simulink model "DigitalShadow"  (R2022a)
settings: Solver=FixedStepDiscrete  StartTime=0.0  StopTime=4  FixedStep=ControlPeriod/10  MaxStep=ControlPeriod/10  RelTol=1e-3
InitFcn:
  | Emrax_params;
model workspace (MAT data in the model file):
  CTRLPERIOD = 5e-05
  TSAMPLE = 2e-06
  global_CLK_number = 0
  global_INT_number = 1
  global_SVM_instance_id = 0
  global_can_baud_rate = '1000000'
  global_comp_time = 0.2
  global_cycle_delay = 0
  global_ip_addresses = {'10.10.10.110', '10.10.10.111', '10.10.10.112', '10.10.10.113'}
values from neighbouring files (symbols this model uses):
  ControlPeriod = 1/ControlFreq    (= 5e-05)    [Emrax_params.m]
  fc_s = 5    [Emrax_params.m]
  PI_d = pidtune(Hd,'PI',2*pi*f_i,opts)    [Emrax_params.m]
  PI_q = pidtune(Hq,'PI',2*pi*f_i,opts)    [Emrax_params.m]
  PI_s = pidtune(Hs,'PI',2*pi*fc_s,opts)    [Emrax_params.m]
  Vdc0 = 400    [Emrax_params.m]
undefined symbols (not defined in the file or in its folder): DiscIntNeverNeededParam, Pmsm
libraries: spsPWMGenerator2LevelLib x3, simulink x2, BoomBox x1, spsabctodq0Lib x1, spsdq0toabcLib x1, spsCurrentMeasurementLib x1, spsDCVoltageSourceLib x1, spsPermanentMagnetSynchronousMachineLib x1, spsThreePhaseSeriesRLCBranchLib x1, spsThreePhaseVIMeasurementLib x1, spsUniversalBridgeLib x1, spsVoltageMeasurementLib x1
settings Model: TunableVars=MODE  TunableVarsStorageClass=ImportedExtern  Creator=imperix  LastModifiedBy=JHANNUM
settings SolverCC: AlgebraicLoopSolver=TrustRegion
settings DataIOCC: LimitDataPoints=on  SaveFormat=Array  SaveOutput=off  SaveTime=off  ReturnWorkspaceOutputs=off
settings OptimizationCC: DefaultUnderspecifiedDataType=single  EnhancedBackFolding=on  PassReuseOutputArgsAs=Individual arguments  ZeroExternalMemoryAtStartup=off  ZeroInternalMemoryAtStartup=off  LifeSpan=inf  SimCompilerOptimization=on  EfficientTunableParamExpr=on
settings DebuggingCC: UnderspecifiedInitializationDetection=Classic  InheritedTsInSrcMsg=none  ParameterPrecisionLossMsg=none  ParameterTunabilityLossMsg=error  UnconnectedInputMsg=warning  UnconnectedOutputMsg=warning  UnconnectedLineMsg=warning  SFUnexpectedBacktrackingDiag=warning  SFNoUnconditionalDefaultTransitionDiag=warning  SFMachineParentedDataDiag=warning  ArithmeticOperatorsInVariantConditions=warning
settings HardwareCC: ProdBitPerPointer=32  ProdBitPerSizeT=32  ProdBitPerPtrDiffT=32  ProdLargestAtomicInteger=Long  ProdLargestAtomicFloat=Double  ProdWordSize=32  ProdHWDeviceType=ARM Compatible->ARM Cortex
settings ModelReferenceCC: UpdateModelReferenceTargets=IfOutOfDate  PropagateSignalLabelsOutOfModel=off
settings SFSimCC: SFSimEcho=off  SimUseLocalCustomCode=off  MATLABDynamicMemAlloc=off  CustomCodeUndefinedFunction=UseInterfaceOnly  SimTargetLang=C++
settings RTWCC: Description=Embedded Coder for imperix products  SystemTargetFile=imperix_ACG_SDK.tlc  TemplateMakefile=imperix_ACG_SDK.tmf  RTWUseLocalCustomCode=off  RTWUseSimCustomCode=on  TargetLang=C++  RTWCustomCompilerOptimizations=-a  DLArmComputeVersion=19.05
settings CodeAppCC: ForceParamTrailComments=on  IgnoreCustomStorageClasses=off  OperatorAnnotations=on  SimulinkDataObjDesc=on  SFDataObjDesc=on  InsertBlockDesc=on  StateflowObjectComments=on
settings STFCustomTargetCC: MultiwordLength=256  ModelReferenceCompliant=off  CombineOutputUpdateFcns=on  ERTCustomFileBanners=on  SupportContinuousTime=off  SupportNonInlinedSFcns=off  RemoveResetFunc=on  MATLABClassNameForMDSCustomization=Simulink.SoftwareTarget.ERTCustomization  GRTInterface=off  SystemTargetFile=imperix_ACG_SDK.tlc
settings ERTTargetCC: ModelReferenceCompliant=off  ParMdlRefBuildCompliant=off  CompOptLevelCompliant=off  ConcurrentExecutionCompliant=off  ModelStepFunctionPrototypeControlCompliant=off  CPPClassGenCompliant=off  UseToolchainInfoCompliant=off  ExtModeStaticAlloc=on  ExtModeStaticAllocSize=100000  ERTSrcFileBannerTemplate=imperix_ACG_SDK_code_template.cgt  ERTHdrFileBannerTemplate=imperix_ACG_SDK_code_template.cgt  ERTDataSrcFileTemplate=imperix_ACG_SDK_code_template.cgt  ERTDataHdrFileTemplate=imperix_ACG_SDK_code_template.cgt  ERTCustomFileTemplate=imperix_ACG_SDK_file_process.tlc  MemSecPackage=Simulink
settings ConfigComp: CovMetricSettings=dw  CovSaveCumulativeToWorkspaceVar=on  CovSaveSingleToWorkspaceVar=on  CovExternalEMLEnable=off
settings SimscapeCC: SimscapeNormalizeSystem=off

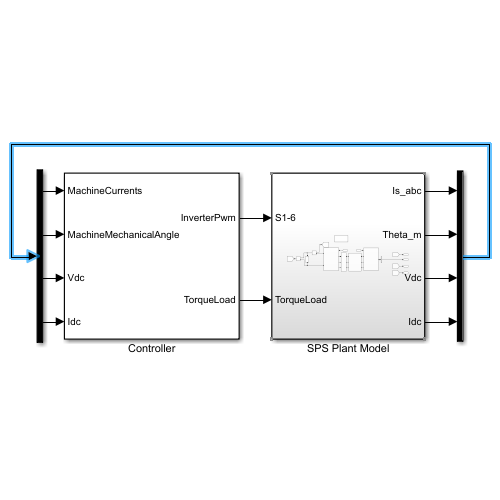
[thumbnail: Simulink's stored preview of the top-level diagram]
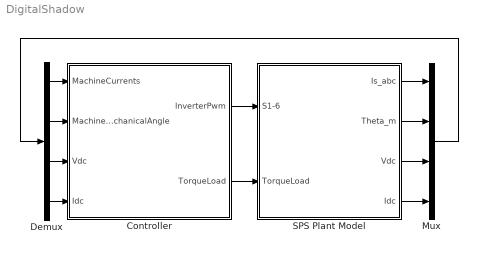
== system DigitalShadow ==
  Controller : Subsystem
  Demux : Demux  Outputs=[3 1 1 1]
  Mux : Mux  Inputs=[3 1 1 1]
  SPS Plant Model : Subsystem
  wires:
  Controller/1(InverterPwm) -> SPS Plant Model/1(S1-6)
  Demux/2 -> Controller/2(MachineMechanicalAngle)
  SPS Plant Model/2(Theta_m) -> Mux/2
  Demux/1 -> Controller/1(MachineCurrents)
  SPS Plant Model/1(Is_abc) -> Mux/1
  SPS Plant Model/3(Vdc) -> Mux/3
  SPS Plant Model/4(Idc) -> Mux/4
  Demux/3 -> Controller/3(Vdc)
  Demux/4 -> Controller/4(Idc)
  Mux/1 -> Demux/1
  Controller/2(TorqueLoad) -> SPS Plant Model/2(TorqueLoad)

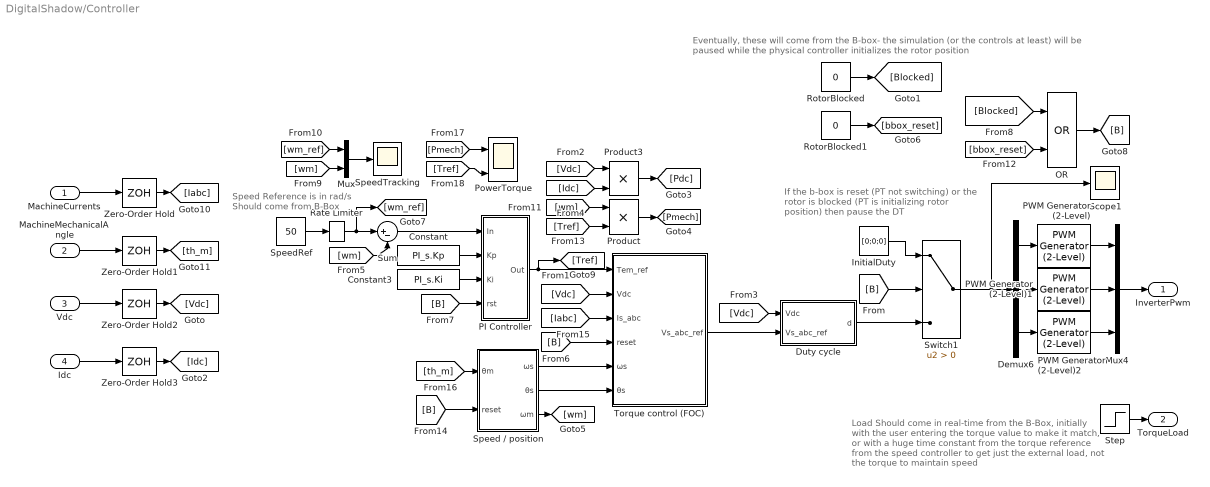
== system DigitalShadow/Controller ==
  note: Speed Reference is in rad/s
      | Should come from B-Box
  note: If the b-box is reset (PT not switching) or the rotor is blocked (PT is initializing rotor position) then pause the DT
  note: Eventually, these will come from the B-box- the simulation (or the controls at least) will be paused while the physical controller initializes the rotor position
  note: Load Should come in real-time from the B-Box, initially with the user entering the torque value to make it match, or with a huge time constant from the torque reference from the speed controller to get just the external load, not the torque to maintain speed
  MachineCurrents : Inport
  MachineMechanicalAngle : Inport  Port=2
  Vdc : Inport  Port=3
  Idc : Inport  Port=4
  Constant : Constant  Value=PI_s.Kp  SampleTime=ControlPeriod
  Constant3 : Constant  Value=PI_s.Ki  SampleTime=ControlPeriod
  Demux6 : Demux  Outputs=3
  Duty cycle : Subsystem
  InitialDuty : Constant  Value=[0;0;0]  SampleTime=ControlPeriod
  Mux : Mux  Inputs=2
  Mux4 : Mux  Inputs=3
  OR : Logic  Operator=OR  IconShape=distinctive  AllPortsSameDT=off  OutDataTypeStr=boolean
  PI Controller : Subsystem  mask(PI controller){I_MODE=Trapezoidal, SamplingTime=ControlPeriod, S_MODE=on, SaturationUpperLimit=100, SaturationLowerLimit=-100, LinearizeAsGain=off, ANTI_WINDUP=back-calculation, K_B=0.1*sqrt(PI_s.Kp*PI_s.Ki)}
      mask prompts: S_MODE "Limit output"; LinearizeAsGain "Ignore saturation when linearizing"
      mask help: This subsystem implements a Proportional Integral (PI) controller, as described in the Technical Note T105.
      mask init:
      | thisBlock = gcb;
      | 
      | 
      | 
      | % change the integrator mode depending on the radio button
      | tempBlock = [gcb '/Integrator'];
      | int_mode = get_param(thisBlock, 'I_MODE')
      | if strcmp('Forward Euler', int_mode)
      |     set_param(tempBlock,'IntegratorMethod','Integration: Forward Euler' )  
      | elseif strcmp('Backward Euler', int_mode)
      |     set_param(tempBlock,'IntegratorMethod','Integration: Backward Euler')  
      | else
      |     set_param(tempBlock,'IntegratorMethod','Integration: Trapezoidal' )  
      | end
      | 
      | 
      | % change the parameters in the saturation block
      | tempBlock = [gcb '/Saturation'];
      | if strcmp('on', get_param(gcb, 'S_MODE'))
      |     set_param(tempBlock, 'OverrideUsingVariant', 'WITH_SATURATION'); 
      | else
      |     set_param(tempBlock, 'OverrideUsingVariant', 'WITHOUT_SATURATION'); 
      | end
      | tempBlock = [gcb '/Saturation/With saturation/Saturation'];
      | set_param(tempBlock, 'UpperLimit', get_param(thisBlock, 'SaturationUpperLimit')); 
      | set_param(tempBlock, 'LowerLimit', get_param(thisBlock, 'SaturationLowerLimit')); 
      | set_param(tempBlock, 'LinearizeAsGain', get_param(thisBlock, 'LinearizeAsGain')); 
      | 
      | 
      | 
      | % change the anti-windup
      | tempBlock = [gcb '/Anti-windup'];
      | if strcmp('none', get_param(thisBlock, 'ANTI_WINDUP'))
      |     set_param(tempBlock, 'OverrideUsingVariant', 'WITHOUT_ANTI_WINDUP'); 
      | else
      |     set_param(tempBlock, 'OverrideUsingVariant', 'WITH_ANTI_WINDUP'); 
      | end
      | tempBlock = [gcb '/Anti-windup/With anti-windup/Kb'];
      | set_param(tempBlock, 'Gain', get_param(thisBlock, 'K_B')); 
      | 
      | clear thisBlock tempBlock
      mask TypeOptions I_MODE: Forward Euler | Backward Euler | Trapezoidal
      mask Callback I_MODE:
      | thisBlock = gcb;
      | tempBlock = [gcb '/Integrator'];
      | 
      | % change the integrator mode depending on the radio button:
      | int_mode = get_param(thisBlock, 'I_MODE')
      | if strcmp('Forward Euler', int_mode)
      |     set_param(tempBlock,'IntegratorMethod','Integration: Forward Euler' )
      | elseif strcmp('Backward Euler', int_mode)
      |     set_param(tempBlock,'IntegratorMethod','Integration: Backward Euler')
      | else
      |     set_param(tempBlock,'IntegratorMethod','Integration: Trapezoidal' )
      | end
      | 
      | clear thisBlock tempBlock;
      mask Callback S_MODE:
      | thisBlock = gcb;
      | tempBlock = [gcb '/Saturation'];
      | 
      | % change the saturation mode depending on the radio button:
      | if strcmp('on', get_param(gcb, 'S_MODE'))
      |     set_param(tempBlock, 'OverrideUsingVariant', 'WITH_SATURATION');
      | else
      |     set_param(tempBlock, 'OverrideUsingVariant', 'WITHOUT_SATURATION');
      | end
      | 
      | % Hide or show parameters
      | maskNames = get_param(thisBlock, 'MaskNames');
      | maskEnable = get_param(thisBlock, 'MaskEnables');
      | 
      | if strcmp(get_param(thisBlock, 'S_MODE'),'on')
      |     %show parameters
      |     maskEnable{strmatch('SaturationUpperLimit',  maskNames, 'exact')} = 'on';
      |     maskEnable{strmatch('SaturationLowerLimit',   maskNames, 'exact')} = 'on';
      |     maskEnable{strmatch('LinearizeAsGain',   maskNames, 'exact')} = 'on';
      |     maskEnable{strmatch('ANTI_WINDUP',   maskNames, 'exact')} = 'on';
      |     maskEnable{strmatch('K_B',   maskNames, 'exact')} = 'on';
      | else
      |     %hide parameters
      |     maskEnable{strmatch('SaturationUpperLimit',  maskNames, 'exact')} = 'off';
      |     maskEnable{strmatch('SaturationLowerLimit',   maskNames, 'exact')} = 'off';
      |     maskEnable{strmatch('LinearizeAsGain',   maskNames, 'exact')} = 'off';
      |     maskEnable{strmatch('ANTI_WINDUP',   maskNames, 'exact')} = 'off';
      |     maskEnable{strmatch('K_B',   maskNames, 'exact')} = 'off';
      | end
      | 
      | set_param(thisBlock, 'MaskEnables', maskEnable);
      | 
      | clear thisBlock tempBlock maskNames maskEnable;
      mask Callback SaturationUpperLimit:
      | thisBlock = gcb;
      | tempBlock = [gcb '/Saturation/With saturation/Saturation'];
      | 
      | % change the parameter in the subblock
      | set_param(tempBlock, 'UpperLimit', get_param(thisBlock, 'SaturationUpperLimit'));
      | 
      | clear thisBlock tempBlock
      mask Callback SaturationLowerLimit:
      | thisBlock = gcb;
      | tempBlock = [gcb '/Saturation/With saturation/Saturation'];
      | 
      | % change the parameter in the subblock
      | set_param(tempBlock, 'LowerLimit', get_param(thisBlock, 'SaturationLowerLimit'));
      | 
      | clear thisBlock tempBlock
      mask Callback LinearizeAsGain:
      | thisBlock = gcb;
      | tempBlock = [gcb '/Saturation/With saturation/Saturation'];
      | 
      | % change the parameter in the subblock
      | set_param(tempBlock, 'LinearizeAsGain', get_param(thisBlock, 'LinearizeAsGain'));
      | 
      | clear thisBlock tempBlock
      mask TypeOptions ANTI_WINDUP: none | back-calculation
      mask Callback ANTI_WINDUP:
      | thisBlock = gcb;
      | tempBlock = [gcb '/Anti-windup'];
      | 
      | % change the saturation mode depending on the radio button:
      | if strcmp('none', get_param(thisBlock, 'ANTI_WINDUP'))
      |     set_param(tempBlock, 'OverrideUsingVariant', 'WITHOUT_ANTI_WINDUP');
      | else
      |     set_param(tempBlock, 'OverrideUsingVariant', 'WITH_ANTI_WINDUP');
      | end
      | 
      | % Hide or show parameters
      | maskNames = get_param(thisBlock, 'MaskNames');
      | MaskVisibility = get_param(thisBlock, 'MaskVisibilities');
      | 
      | if strcmp(get_param(thisBlock, 'ANTI_WINDUP'),'none')
      |     %hide parameters
      |     MaskVisibility{strmatch('K_B',  maskNames, 'exact')} = 'off';
      |     %thisBlock.getDialogControl('KBtext').Visible='off';
      | else
      |     %show parameters
      |     MaskVisibility{strmatch('K_B',  maskNames, 'exact')} = 'on';
      |     %thisBlock.getDialogControl('KBtext').Visible='on';
      | end
      | 
      | set_param(thisBlock, 'MaskVisibilities', MaskVisibility);
      | 
      | clear thisBlock tempBlock maskNames MaskVisibility;
      mask Callback K_B:
      | thisBlock = gcb;
      | tempBlock = [gcb '/Anti-windup/With anti-windup/Kb'];
      | 
      | % change the parameter in the subblock
      | set_param(tempBlock, 'Gain', get_param(thisBlock, 'K_B'));
      | 
      | clear thisBlock tempBlock
      mask DialogControl DiscreteText Prompt: Discrete-time settings
      mask DialogControl I_MODEText Prompt: Integrator method:
      mask DialogControl SamplingTimeText Prompt: Sample time (-1 for inherited)
      mask DialogControl SaturationText Prompt: Output saturation
      mask DialogControl Control4 Prompt: Upper saturation limit:
      mask DialogControl Control5 Prompt: Lower saturation limit:
      mask DialogControl Control6 Prompt: Anti-windup method:
      mask DialogControl KBtext Prompt: Back-calculation coefficient (Kb):
  PWM Generator (2-Level) : spsPWMGenerator2LevelLib/PWM Generator (2-Level)  ModulatorType=Single-phase half-bridge (2 pulses)  ModulatorMode=Unsynchronized  Fc=ControlFreq  Pc=0  nF=1  MinMax=[0 1]  SamplingTechnique=Symmetrical regular (single edge)  ModulatingSignals=off  m=0.8  Freq=60  Phase=0  Ts=ControlPeriod/10  ShowCarrierOutport=off
  PWM Generator (2-Level)1 : spsPWMGenerator2LevelLib/PWM Generator (2-Level)  ModulatorType=Single-phase half-bridge (2 pulses)  ModulatorMode=Unsynchronized  Fc=ControlFreq  Pc=0  nF=1  MinMax=[0 1]  SamplingTechnique=Symmetrical regular (single edge)  ModulatingSignals=off  m=0.8  Freq=60  Phase=0  Ts=ControlPeriod/10  ShowCarrierOutport=off
  PWM Generator (2-Level)2 : spsPWMGenerator2LevelLib/PWM Generator (2-Level)  ModulatorType=Single-phase half-bridge (2 pulses)  ModulatorMode=Unsynchronized  Fc=ControlFreq  Pc=0  nF=1  MinMax=[0 1]  SamplingTechnique=Symmetrical regular (single edge)  ModulatingSignals=off  m=0.8  Freq=60  Phase=0  Ts=ControlPeriod/10  ShowCarrierOutport=off
  PowerTorque : Scope  NumInputPorts=2
  Product : Product
  Product3 : Product
  Rate Limiter : RateLimiter  RisingSlewLimit=100  FallingSlewLimit=-25  SampleTimeMode=inherited  LinearizeAsGain=off
  RotorBlocked : Constant  Value=0  SampleTime=ControlPeriod
  RotorBlocked1 : Constant  Value=0  SampleTime=ControlPeriod
  Scope1 : Scope
  Speed / position : Subsystem
  SpeedRef : Constant  Value=50  SampleTime=ControlPeriod
  SpeedTracking : Scope
  Step : Step  After=10  SampleTime=ControlPeriod
  Sum : Sum  Inputs=|+-
  Switch1 : Switch  Criteria=u2 > Threshold  SaturateOnIntegerOverflow=off  InputSameDT=off
  Torque control (FOC) : Subsystem
  Zero-Order Hold{,1..3} (4 alike) : ZeroOrderHold  SampleTime=ControlPeriod
  InverterPwm : Outport
  TorqueLoad : Outport  Port=2
  wires:
  PWM Generator (2-Level)1/1 -> Mux4/2
  PWM Generator (2-Level)/1 -> Mux4/1
  PWM Generator (2-Level)2/1 -> Mux4/3
  [Vdc] -> Torque control (FOC)/2(Vdc)
  Speed / position/2(θs) -> Torque control (FOC)/6(θs)
  Torque control (FOC)/1(Vs_abc_ref) -> Duty cycle/2(Vs_abc_ref)
  [Vdc] -> Duty cycle/1(Vdc)
  Sum/1 -> PI Controller/1(In)
  Speed / position/3(" ωm") -> [wm]
  Mux4/1 -> InverterPwm/1
  Duty cycle/1(d) -> Switch1/3
  Switch1/1 -> Scope1/1, Demux6/1
  [B] -> Switch1/2
  PI Controller/1(Out) -> Torque control (FOC)/1(Tem_ref), [Tref]
  [B] -> Torque control (FOC)/4(reset)
  [B] -> PI Controller/4(rst)
  Rate Limiter/1 -> [wm_ref], Sum/1
  [B] -> Speed / position/2(reset)
  Speed / position/1(" ωs") -> Torque control (FOC)/5(ωs)
  Product/1 -> [Pmech]
  [Vdc] -> Product3/1
  [Idc] -> Product3/2
  Product3/1 -> [Pdc]
  SpeedRef/1 -> Rate Limiter/1
  Demux6/3 -> PWM Generator (2-Level)2/1
  Demux6/1 -> PWM Generator (2-Level)/1
  Demux6/2 -> PWM Generator (2-Level)1/1
  [wm] -> Sum/2
  Constant3/1 -> PI Controller/3(Ki)
  Constant/1 -> PI Controller/2(Kp)
  [wm] -> Mux/2
  [wm_ref] -> Mux/1
  Mux/1 -> SpeedTracking/1
  [wm] -> Product/1
  InitialDuty/1 -> Switch1/1
  RotorBlocked1/1 -> [bbox_reset]
  [Blocked] -> OR/1
  [bbox_reset] -> OR/2
  OR/1 -> [B]
  [Tref] -> Product/2
  [Iabc] -> Torque control (FOC)/3(Is_abc)
  [th_m] -> Speed / position/1(θm)
  Zero-Order Hold/1 -> [Iabc]
  Zero-Order Hold1/1 -> [th_m]
  Zero-Order Hold2/1 -> [Vdc]
  Zero-Order Hold3/1 -> [Idc]
  RotorBlocked/1 -> [Blocked]
  [Pmech] -> PowerTorque/1
  [Tref] -> PowerTorque/2
  MachineCurrents/1 -> Zero-Order Hold/1
  MachineMechanicalAngle/1 -> Zero-Order Hold1/1
  Vdc/1 -> Zero-Order Hold2/1
  Idc/1 -> Zero-Order Hold3/1
  Step/1 -> TorqueLoad/1

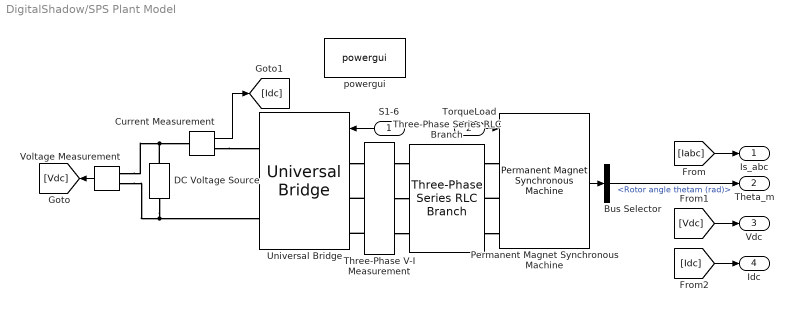
== system DigitalShadow/SPS Plant Model ==
  S1-6 : Inport
  TorqueLoad : Inport  Port=2
  Bus Selector : BusSelector  OutputSignals=Rotor angle thetam (rad)
  Current Measurement : spsCurrentMeasurementLib/Current Measurement  PhasorSimulation=off  OutputType=Complex  PSBequivalent=0
  DC Voltage Source : spsDCVoltageSourceLib/DC Voltage Source  Amplitude=Vdc0  Measurements=None
  Permanent Magnet Synchronous Machine : spsPermanentMagnetSynchronousMachineLib/Permanent Magnet Synchronous Machine  NbPhases=3  FluxDistribution=Sinusoidal  RotorType=Salient-pole  MechanicalLoad=Torque Tm  PresetModel=No  ShowDetailedParameters=on  MeasurementBus=off  Resistance=Pmsm.Rs  Inductance=8.5e-3  dqInductances=[76e-6,79e-6]  La=0.000395  MachineConstant=Flux linkage established by magnets (V.s)  Flux=Pmsm.Phi_pm  VoltageCst=64.3899  TorqueCst=0.5325  Flat=120  Mechanical=[Pmsm.Jm 0 Pmsm.p 0]  PolePairs=4  InitialConditions=[0,0, 0,0]  InitialConditions5ph=[0 0 0 0 0 0]  RefAngle=Aligned with phase A axis (original Park)  IterativeDiscreteModel=Trapezoidal robust  TsBlock=ControlPeriod/100  TsPowergui=0
  Three-Phase Series RLC Branch : spsThreePhaseSeriesRLCBranchLib/Three-Phase Series RLC Branch  LConnTagsString=A|B|C  RConnTagsString=A|B|C  BranchType=L  Resistance=1  Inductance=Pmsm.Lext  Capacitance=1e-6  Measurements=None
  Three-Phase V-I Measurement : spsThreePhaseVIMeasurementLib/Three-Phase V-I Measurement  VoltageMeasurement=phase-to-phase  SetLabelV=on  LabelV=Vabc  Vpu=off  VpuLL=off  CurrentMeasurement=yes  SetLabelI=on  LabelI=Iabc  Ipu=off  Pbase=100e6  Vbase=500e3  OutputType=Complex  PhasorSimulation=off  PSBequivalent=0
  Universal Bridge : spsUniversalBridgeLib/Universal Bridge  Arms=3  SnubberResistance=1e5  SnubberCapacitance=inf  Device=MOSFET / Diodes  Ron=1e-3  Lon=0  ForwardVoltages="[  0  0  ]"  ForwardVoltage=0  GTOparameters=[ 10e-6 , 20e-6 ]  IGBTparameters=[ 1e-6 , 2e-6 ]  Measurements=None  Measurements_2=None  converterType=Rectifier
  Voltage Measurement : spsVoltageMeasurementLib/Voltage Measurement  PhasorSimulation=off  OutputType=Complex  PSBequivalent=0
  powergui : spspowerguiLib/powergui  Priority=1  SimulationMode=Discrete  SampleTime=ControlPeriod/10  frequency=60  Iterations=50  frequencyindice=0  Pbase=100e6  ErrMax=1e-4  UnitsV=kV  UnitsW=MW  buscounter=0  FunctionMessages=off  echomessages=off  EnableUseOfTLC=off  CurrentSourceSwitches=off  DisableSnubberDevices=off  DisableRonSwitches=off  DisableVfSwitches=off  DisplayEquations=off  AutomaticDiscreteSolvers=off  SolverType=Tustin/Backward Euler (TBE)  Interpol=off  ExternalGateDelay=off  methode=off  Ts=100  x0status=blocks  SPID=on  SwTol=0  HookPort=off  NonlinearTolerance=1e-4  nMaxIteration=100  ContinueOnMaxIteration=off  RestoreLinks=warning  ResistiveCurrentMeasurement=off  Frange=[0:2:500]  Ylog=off  Xlog=on  ShowGrid=off  save=off  variable=ZData  structure=0  ZoomFFT=off  StartTime=0.0  cycles=1  DisplayStyle=1  fundamental=60  FreqAxis=off  MaxFrequency=1000  frequencyindicesteady=1  RmsSteady=1  display=off
  Is_abc : Outport
  Theta_m : Outport  Port=2
  Vdc : Outport  Port=3
  Idc : Outport  Port=4
  wires:
  S1-6/1 -> Universal Bridge/1
  [Iabc] -> Is_abc/1
  Voltage Measurement/1 -> [Vdc]
  [Vdc] -> Vdc/1
  Current Measurement/1 -> [Idc]
  [Idc] -> Idc/1
  Permanent Magnet Synchronous Machine/1 -> Bus Selector/1
  Bus Selector/1 -> Theta_m/1  "<Rotor angle thetam (rad)>"
  TorqueLoad/1 -> Permanent Magnet Synchronous Machine/1
  connections:
  DC Voltage Source/LConn1 -- Voltage Measurement/LConn2 -- Universal Bridge/RConn2
  Three-Phase V-I Measurement/LConn3 -- Universal Bridge/LConn3
  Three-Phase V-I Measurement/LConn2 -- Universal Bridge/LConn2
  Universal Bridge/LConn1 -- Three-Phase V-I Measurement/LConn1
  Three-Phase V-I Measurement/RConn3 -- Three-Phase Series RLC Branch/LConn3
  Three-Phase V-I Measurement/RConn2 -- Three-Phase Series RLC Branch/LConn2
  Three-Phase V-I Measurement/RConn1 -- Three-Phase Series RLC Branch/LConn1
  Three-Phase Series RLC Branch/RConn1 -- Permanent Magnet Synchronous Machine/LConn1
  Permanent Magnet Synchronous Machine/LConn2 -- Three-Phase Series RLC Branch/RConn2
  Three-Phase Series RLC Branch/RConn3 -- Permanent Magnet Synchronous Machine/LConn3
  Voltage Measurement/LConn1 -- Current Measurement/LConn1 -- DC Voltage Source/RConn1
  Current Measurement/RConn1 -- Universal Bridge/RConn1

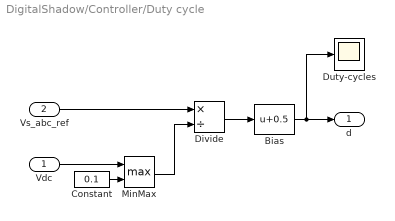
== system DigitalShadow/Controller/Duty cycle ==
  Vdc : Inport
  Vs_abc_ref : Inport  Port=2
  Bias : Bias  Bias=0.5  SaturateOnIntegerOverflow=off
  Constant : Constant  Value=0.1  OutDataTypeStr=single
  Divide : Product  Inputs=*/
  Duty-cycles : Scope
  MinMax : MinMax  Function=max  Inputs=2
  d : Outport
  wires:
  Vs_abc_ref/1 -> Divide/1
  Vdc/1 -> MinMax/1
  MinMax/1 -> Divide/2
  Constant/1 -> MinMax/2
  Divide/1 -> Bias/1
  Bias/1 -> Duty-cycles/1, d/1

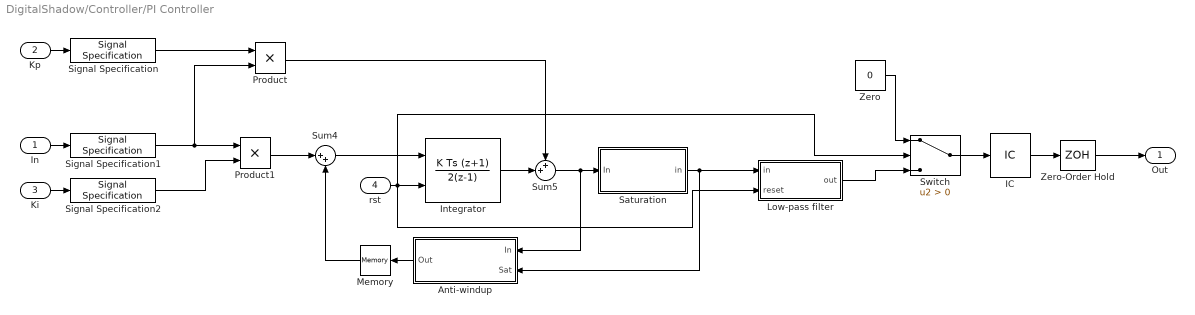
== system DigitalShadow/Controller/PI Controller ==
  In : Inport
  Kp : Inport  Port=2
  Ki : Inport  Port=3
  rst : Inport  Port=4
  Anti-windup : Subsystem  Variant=on  VariantControlMode=label  LabelModeActiveChoice=WITH_ANTI_WINDUP
  IC : InitialCondition  Value=0
  Integrator : DiscreteIntegrator  IntegratorMethod=Integration: Trapezoidal  ExternalReset=level  SampleTime=SamplingTime  ICPrevOutput=DiscIntNeverNeededParam  ICPrevScaledInput=DiscIntNeverNeededParam
  Low-pass filter : Subsystem
  Memory : Memory
  Product : Product
  Product1 : Product
  Saturation : Subsystem  Variant=on  VariantControlMode=label  LabelModeActiveChoice=WITH_SATURATION
  Signal Specification : SignalSpecification  SampleTime=SamplingTime
  Signal Specification1 : SignalSpecification  SampleTime=SamplingTime
  Signal Specification2 : SignalSpecification  SampleTime=SamplingTime
  Sum4 : Sum  Inputs=|++
  Sum5 : Sum  Inputs=++|
  Switch : Switch  Criteria=u2 > Threshold  SaturateOnIntegerOverflow=off  InputSameDT=off
  Zero : Constant  Value=0  OutDataTypeStr=Inherit: Inherit via back propagation
  Zero-Order Hold : ZeroOrderHold  SampleTime=CTRLPERIOD
  Out : Outport
  wires:
  Signal Specification2/1 -> Product1/2
  Signal Specification1/1 -> Product/2, Product1/1
  Signal Specification/1 -> Product/1
  Saturation/1(in) -> Low-pass filter/1(in), Anti-windup/2(Sat)
  Sum4/1 -> Integrator/1
  Kp/1 -> Signal Specification/1
  Product/1 -> Sum5/1
  Product1/1 -> Sum4/1
  Integrator/1 -> Sum5/2
  rst/1 -> Integrator/2, Low-pass filter/2(reset), Switch/2
  Sum5/1 -> Saturation/1(In), Anti-windup/1(In)
  In/1 -> Signal Specification1/1
  Ki/1 -> Signal Specification2/1
  Anti-windup/1(Out) -> Memory/1
  Memory/1 -> Sum4/2
  Switch/1 -> IC/1
  Zero/1 -> Switch/1
  IC/1 -> Zero-Order Hold/1
  Zero-Order Hold/1 -> Out/1
  Low-pass filter/1(out) -> Switch/3

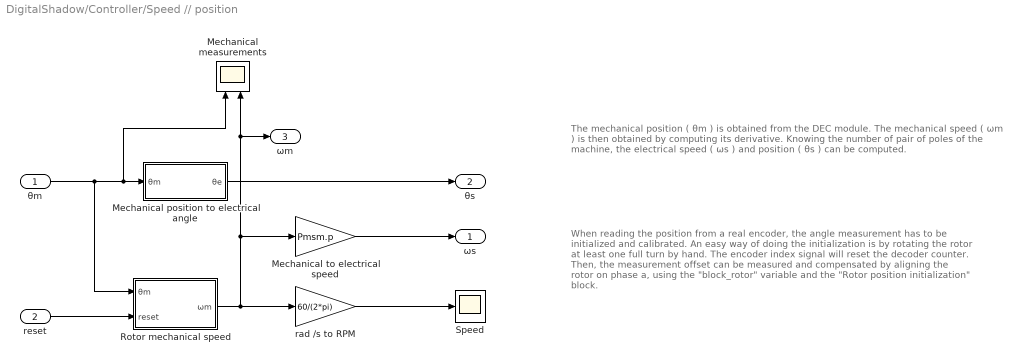
== system DigitalShadow/Controller/Speed // position ==
  note: The mechanical position ( θm ) is obtained from the DEC module.
      |
      | The mechanical speed ( ωm ) is then obtained by computing its derivative.
      |
      | Knowing the number of pair of poles of the machine, the electrical speed ( ωs ) and position ( θs ) can be computed.
  note: When reading the position from a real encoder, the angle measurement has to be initialized and calibrated.
      |
      | An easy way of doing the initialization is by rotating the rotor at least one full turn by hand. The encoder index signal will reset the decoder counter.
      |
      | Then, the measurement offset can be measured and compensated by aligning the rotor on phase a, using the "block_rotor" variable and the "Rotor position initialization" block.
  θm : Inport
  reset : Inport  Port=2
  Mechanical measurements : Scope  NumInputPorts=2
  Mechanical position to electrical angle : Subsystem  mask{p=Pmsm.p}
      mask prompts: p "Number of pole pairs"
  Mechanical to electrical speed : Gain  Gain=Pmsm.p
  Rotor mechanical speed : Subsystem  mask{fc=100}
      mask prompts: fc "Filter cutoff frequency [Hz]"
      mask help:
      | The rotor speed is obtained by differentiation of the measured angle. The "function block" removes angle discontinuities.
      |
      | The derivative is then filtered to reduce the noise introduced by the numerical differentiation.
      |
      | Additional details can be found in "PN104: Using the angle decoder modules" on the imperix knowledge base (kb.imperix.com).
  Speed : Scope
  rad /s to RPM : Gain  Gain=60/(2*pi)
  " ωs" : Outport
  θs : Outport  Port=2
  " ωm" : Outport  Port=3
  wires:
  reset/1 -> Rotor mechanical speed/2(reset)
  Mechanical position to electrical angle/1(θe) -> θs/1
  θm/1 -> Rotor mechanical speed/1(θm), Mechanical measurements/1, Mechanical position to electrical angle/1(θm)
  Rotor mechanical speed/1(ωm) -> rad /s to RPM/1, Mechanical to electrical speed/1, " ωm"/1, Mechanical measurements/2
  rad /s to RPM/1 -> Speed/1
  Mechanical to electrical speed/1 -> " ωs"/1

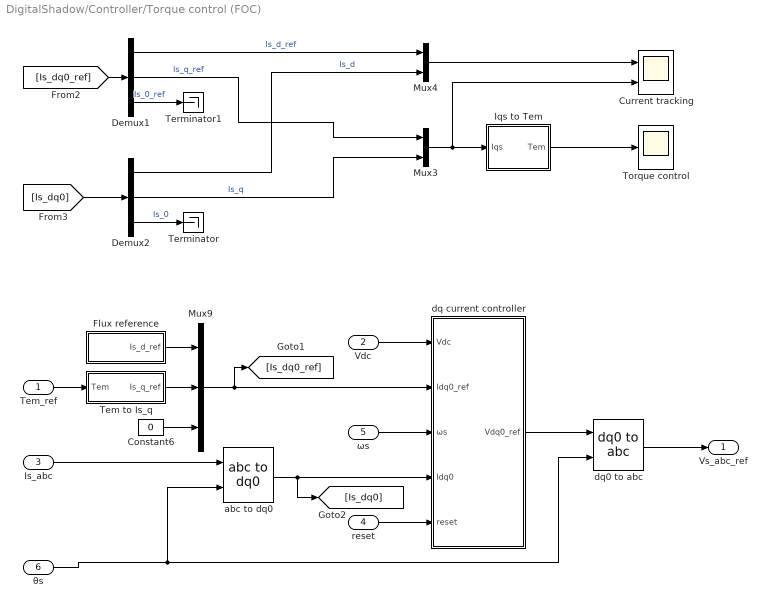
== system DigitalShadow/Controller/Torque control (FOC) ==
  Tem_ref : Inport
  Vdc : Inport  Port=2
  Is_abc : Inport  Port=3
  reset : Inport  Port=4
  ωs : Inport  Port=5
  θs : Inport  Port=6
  Constant6 : Constant  Value=0  OutDataTypeStr=Inherit: Inherit via back propagation
  Current tracking : Scope  NumInputPorts=2
  Demux1 : Demux  Outputs=3
  Demux2 : Demux  Outputs=3
  Flux reference : Subsystem
  Iqs to Tem : Subsystem  mask{p=Pmsm.p, Phi_pm=Pmsm.Phi_pm}
      mask prompts: p "Number of pole pairs"; Phi_pm "Magnets flux"
  Mux3 : Mux  Inputs=2
  Mux4 : Mux  Inputs=2
  Mux9 : Mux  Inputs=[1 1 1]
  Tem to Is_q : Subsystem  mask{p=Pmsm.p, Phi_pm=Pmsm.Phi_pm}
      mask prompts: p "Number of pole pairs"; Phi_pm "Permanent magnet flux [Wb]"
  Terminator : Terminator
  Terminator1 : Terminator
  Torque control : Scope
  abc to dq0 : spsabctodq0Lib/abc to dq0  Alignment=Aligned with phase A axis
  dq current controller : Subsystem  mask{Ld=Pmsm.Ld, Kpd=PI_d.Kp, Kid=PI_d.Ki, Lq=Pmsm.Lq, Kpq=PI_q.Kp, Kiq=PI_q.Ki}
      mask prompts: Ld "Inductance Ld"; Kpd "Proportional gain Kp"; Kid "Integral gain Ki"; Lq "Inductance Lq"; Kpq "Proportional gain Kp"; Kiq "Integral gain Ki"
      mask DialogControl ParameterGroupVar Prompt: Parameters: d-axis
      mask DialogControl Container3 Prompt: Parameters: q-axis
  dq0 to abc : spsdq0toabcLib/dq0 to abc  Alignment=Aligned with phase A axis
  Vs_abc_ref : Outport
  wires:
  Tem_ref/1 -> Tem to Is_q/1(Tem)
  Tem to Is_q/1(Is_q_ref) -> Mux9/2
  Flux reference/1(Is_d_ref) -> Mux9/1
  Constant6/1 -> Mux9/3
  dq0 to abc/1 -> Vs_abc_ref/1
  θs/1 -> dq0 to abc/2, abc to dq0/2
  abc to dq0/1 -> dq current controller/4(Idq0), [Is_dq0]
  reset/1 -> dq current controller/5(reset)
  Mux9/1 -> dq current controller/2(Idq0_ref), [Is_dq0_ref]
  dq current controller/1(Vdq0_ref) -> dq0 to abc/1
  Is_abc/1 -> abc to dq0/1
  Vdc/1 -> dq current controller/1(Vdc)
  Demux2/3 -> Terminator/1  "Is_0"
  Demux2/1 -> Mux4/2  "Is_d"
  Demux2/2 -> Mux3/2  "Is_q"
  Mux3/1 -> Current tracking/2, Iqs to Tem/1(Iqs)
  Mux4/1 -> Current tracking/1
  Iqs to Tem/1(Tem) -> Torque control/1
  Demux1/3 -> Terminator1/1  "Is_0_ref"
  Demux1/1 -> Mux4/1  "Is_d_ref"
  Demux1/2 -> Mux3/1  "Is_q_ref"
  [Is_dq0] -> Demux2/1
  [Is_dq0_ref] -> Demux1/1
  ωs/1 -> dq current controller/3(ωs)

== system DigitalShadow/Controller/PI Controller/Anti-windup ==
  In : Inport
  Sat : Inport  Port=2
  With anti-windup : Subsystem  VariantControl=WITH_ANTI_WINDUP
  Without anti-windup : Subsystem  VariantControl=WITHOUT_ANTI_WINDUP
  Out : Outport

== system DigitalShadow/Controller/PI Controller/Low-pass filter ==
  note: fc = cut-off frequency (from mask)
      | Ts = sample time
      | tc = 1 / (2*pi*fc);
      | alpha = Ts / (tc + Ts);
  in : Inport
  reset : Inport  Port=2
  Compute alpha : Subsystem
  IIR : Subsystem  mask(Basic IIR LPF filter){}
      mask help:
      | The output is computed as:
      | y[k] = G * y[k-1] + (1-G) * u[k]
  Tunable parameter : BoomBox/Tunable parameter  VARNAME=fc_speed_filter  INITIALVAL=10*fc_s  DATA_TYPE=single  VAL_MAX=Inf  VAL_MIN=-Inf  CAN_ENABLED=off  CAN_ADDRESS=0  can_endianness=Little-endian  init_baudrate=0  CAN_BAUDRATE=1000000  ETH_ENABLED=off  ETH_PORT=2000  eth_endianness=Little-endian  SIM_OUT=Initial value  STEP_TIMES=[0.1 0.2]  STEP_DATA=[1 2]  KBID=kb0501  CAN_BIG_ENDIAN=0  ETH_BIG_ENDIAN=0  CAN_MB_ID=1  ETH_MB_ID=2  RESIZE=0
      settings: SourceProductName=imperix blockset
  out : Outport
  wires:
  in/1 -> IIR/2(u)
  reset/1 -> IIR/3(reset)
  Compute alpha/1(α) -> IIR/1(α)
  IIR/1(y) -> out/1
  Tunable parameter/1 -> Compute alpha/1(fc)

== system DigitalShadow/Controller/PI Controller/Saturation ==
  In : Inport
  With saturation : Subsystem  VariantControl=WITH_SATURATION
  Without saturation : Subsystem  VariantControl=WITHOUT_SATURATION
  in : Outport

== system DigitalShadow/Controller/Speed // position/Mechanical position to electrical angle ==
  note: Converter to electrical rad
  note: Keep mechanical angle
      | in the range [0; pi]
  θm : Inport
  Angle wrapping : Subsystem  Commented=on
  Fcn : Fcn  Expr=u+2*pi*(u < 0)
  Gain : Gain  Gain=p
  θe : Outport
  wires:
  θm/1 -> Fcn/1
  Fcn/1 -> Gain/1
  Gain/1 -> θe/1

== system DigitalShadow/Controller/Speed // position/Rotor mechanical speed ==
  note: The rotor speed is obtained by differentiation of the measured angle. The function block removes angle discontinuities.
      |
      | The derivative is filtered to reduce the noise introduced by the numerical differentiation.
      |
      | See PN104: Using the angle decoder modules
      | on the imperix knowledge base (kb.imperix.com)
  θm : Inport
  reset : Inport  Port=2
  Angle derivator : Subsystem
  Low-pass filter : Subsystem
  ωm : Outport
  wires:
  Low-pass filter/1(out) -> ωm/1
  θm/1 -> Angle derivator/1(angle)
  reset/1 -> Low-pass filter/2(reset)
  Angle derivator/1(speed) -> Low-pass filter/1(in)

== system DigitalShadow/Controller/Torque control (FOC)/Flux reference ==
  note: The d-axis current reference is set to 0A
      | in order to maximize the torque generation.
  Constant : Constant  Value=0  OutDataTypeStr=Inherit: Inherit via back propagation
  Is_d_ref : Outport
  wires:
  Constant/1 -> Is_d_ref/1

== system DigitalShadow/Controller/Torque control (FOC)/Iqs to Tem ==
  Iqs : Inport
  Constant : Constant  Value=1.5*p*Phi_pm  OutDataTypeStr=single
  Product : Product
  Tem : Outport
  wires:
  Constant/1 -> Product/2
  Iqs/1 -> Product/1
  Product/1 -> Tem/1

== system DigitalShadow/Controller/Torque control (FOC)/Tem to Is_q ==
  Tem : Inport
  Constant : Constant  Value=1.5*p*Phi_pm  OutDataTypeStr=Inherit: Inherit via back propagation
  Divide : Product  Inputs=*/
  Is_q_ref : Outport
  wires:
  Constant/1 -> Divide/2
  Tem/1 -> Divide/1
  Divide/1 -> Is_q_ref/1

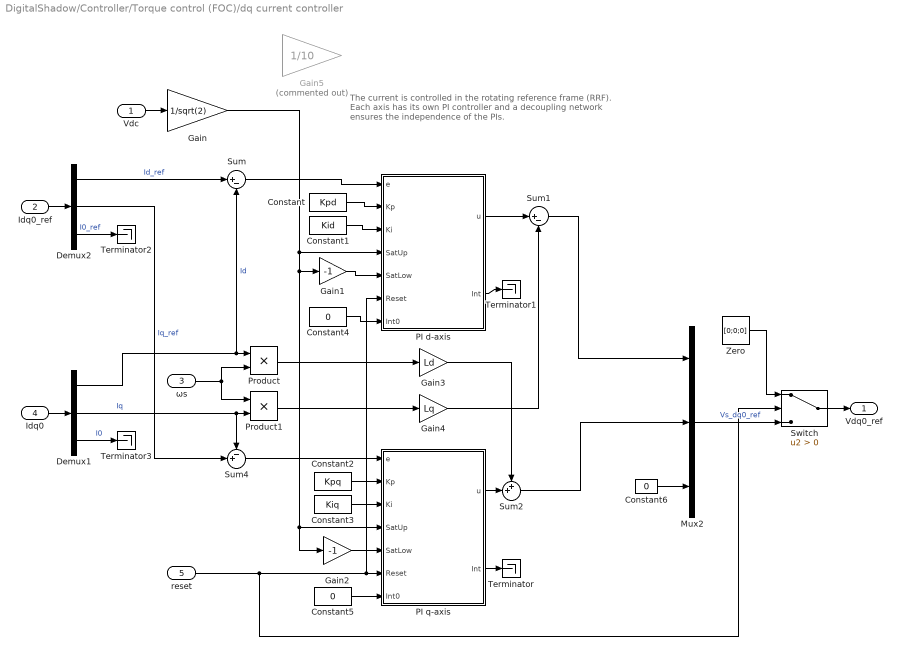
== system DigitalShadow/Controller/Torque control (FOC)/dq current controller ==
  note: The current is controlled in the rotating reference frame (RRF).
      | Each axis has its own PI controller and a decoupling network
      | ensures the independence of the PIs.
  Vdc : Inport
  Idq0_ref : Inport  Port=2
  ωs : Inport  Port=3
  Idq0 : Inport  Port=4
  reset : Inport  Port=5
  Constant : Constant  Value=Kpd  OutDataTypeStr=Inherit: Inherit via back propagation
  Constant1 : Constant  Value=Kid  OutDataTypeStr=Inherit: Inherit via back propagation
  Constant2 : Constant  Value=Kpq  OutDataTypeStr=Inherit: Inherit via back propagation
  Constant3 : Constant  Value=Kiq  OutDataTypeStr=Inherit: Inherit via back propagation
  Constant4 : Constant  Value=0  OutDataTypeStr=Inherit: Inherit via back propagation
  Constant5 : Constant  Value=0  OutDataTypeStr=Inherit: Inherit via back propagation
  Constant6 : Constant  Value=0  OutDataTypeStr=Inherit: Inherit via back propagation
  Demux1 : Demux  Outputs=3
  Demux2 : Demux  Outputs=3
  Gain : Gain  Gain=1/sqrt(2)
  Gain1 : Gain  Gain=-1
  Gain2 : Gain  Gain=-1
  Gain3 : Gain  Gain=Ld
  Gain4 : Gain  Gain=Lq
  Gain5 : Gain  Commented=on  Gain=1/10
  Mux2 : Mux  Inputs=3
  PI d-axis : Subsystem
  PI q-axis : Subsystem
  Product : Product
  Product1 : Product
  Sum : Sum  Inputs=|+-
  Sum1 : Sum  Inputs=|+-
  Sum2 : Sum  Inputs=++|
  Sum4 : Sum  Inputs=-+|
  Switch : Switch  Criteria=u2 > Threshold  OutDataTypeStr=Inherit: Inherit via back propagation  SaturateOnIntegerOverflow=off  InputSameDT=off
  Terminator{,1..3} (4 alike) : Terminator
  Zero : Constant  Value=[0;0;0]  OutDataTypeStr=Inherit: Inherit via back propagation
  Vdq0_ref : Outport
  wires:
  Constant/1 -> PI d-axis/2(Kp)
  Constant1/1 -> PI d-axis/3(Ki)
  Constant3/1 -> PI q-axis/3(Ki)
  Constant2/1 -> PI q-axis/2(Kp)
  Vdc/1 -> Gain/1
  Gain/1 -> Gain2/1, PI q-axis/4(SatUp), Gain1/1, PI d-axis/4(SatUp)
  Gain1/1 -> PI d-axis/5(SatLow)
  Gain2/1 -> PI q-axis/5(SatLow)
  Sum/1 -> PI d-axis/1(e)
  Sum4/1 -> PI q-axis/1(e)
  ωs/1 -> Product/2, Product1/1
  Constant4/1 -> PI d-axis/7(Int0)
  Constant5/1 -> PI q-axis/7(Int0)
  reset/1 -> Switch/2, PI q-axis/6(Reset), PI d-axis/6(Reset)
  Product1/1 -> Gain4/1
  Product/1 -> Gain3/1
  PI d-axis/1(u) -> Sum1/1
  PI q-axis/1(u) -> Sum2/2
  Gain4/1 -> Sum1/2
  PI q-axis/2(Int) -> Terminator/1
  PI d-axis/2(Int) -> Terminator1/1
  Gain3/1 -> Sum2/1
  Demux2/2 -> Sum4/2  "Iq_ref"
  Idq0_ref/1 -> Demux2/1
  Demux2/1 -> Sum/1  "Id_ref"
  Demux2/3 -> Terminator2/1  "I0_ref"
  Demux1/3 -> Terminator3/1  "I0"
  Demux1/1 -> Sum/2, Product/1  "Id"
  Idq0/1 -> Demux1/1
  Demux1/2 -> Sum4/1, Product1/2  "Iq"
  Sum1/1 -> Mux2/1
  Sum2/1 -> Mux2/2
  Constant6/1 -> Mux2/3
  Mux2/1 -> Switch/3  "Vs_dq0_ref"
  Switch/1 -> Vdq0_ref/1
  Zero/1 -> Switch/1

== system DigitalShadow/Controller/PI Controller/Anti-windup/With anti-windup ==
  In : Inport
  Sat : Inport  Port=2
  Kb : Gain  Gain=0.1*sqrt(PI_s.Kp*PI_s.Ki)  SaturateOnIntegerOverflow=on
  Sum : Sum  Inputs=|-+
  Out : Outport
  wires:
  Kb/1 -> Out/1
  Sum/1 -> Kb/1
  In/1 -> Sum/1
  Sat/1 -> Sum/2

== system DigitalShadow/Controller/PI Controller/Anti-windup/Without anti-windup ==
  In : Inport
  Sat : Inport  Port=2
  Terminator : Terminator
  Terminator1 : Terminator
  Out : Outport
  wires:
  Sat/1 -> Terminator1/1
  In/1 -> Terminator/1

== system DigitalShadow/Controller/PI Controller/Low-pass filter/Compute alpha ==
  fc : Inport
  Fcn1 : Fcn  Expr=1/(2*pi*u(1))
  Fcn2 : Fcn  Expr=1/u(1)
  Weighted Sample Time1 : SampleTimeMath
  Weighted Sample Time2 : SampleTimeMath  TsampMathOp=*
  α : Outport
  wires:
  Fcn1/1 -> Weighted Sample Time1/1  "tc"
  fc/1 -> Fcn1/1
  Weighted Sample Time2/1 -> α/1  "Ts/(tc+Ts)"
  Fcn2/1 -> Weighted Sample Time2/1  "1/(tc+Ts)"
  Weighted Sample Time1/1 -> Fcn2/1  "tc+Ts"

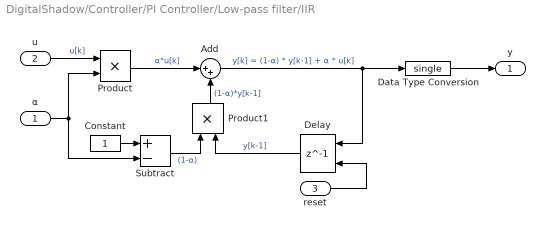
== system DigitalShadow/Controller/PI Controller/Low-pass filter/IIR ==
  α : Inport
  u : Inport  Port=2
  reset : Inport  Port=3
  Add : Sum  Inputs=|++
  Constant : Constant  OutDataTypeStr=Inherit: Inherit via back propagation
  Data Type Conversion : DataTypeConversion  OutDataTypeStr=single  SaturateOnIntegerOverflow=off  RndMeth=Floor
  Delay : Delay  DelayLength=1  ExternalReset=Level hold
      settings: InputPortMap=u0,r5
  Product : Product
  Product1 : Product
  Subtract : Sum  Inputs=+-
  y : Outport
  wires:
  u/1 -> Product/1  "u[k]"
  Subtract/1 -> Product1/1  "(1-α)"
  α/1 -> Subtract/2, Product/2
  Constant/1 -> Subtract/1
  reset/1 -> Delay/2
  Delay/1 -> Product1/2  "y[k-1]"
  Product/1 -> Add/1  "α*u[k]"
  Product1/1 -> Add/2  "(1-α)*y[k-1]"
  Add/1 -> Data Type Conversion/1, Delay/1  "y[k] = (1-α) * y[k-1] + α * u[k]"
  Data Type Conversion/1 -> y/1

== system DigitalShadow/Controller/PI Controller/Saturation/With saturation ==
  In : Inport
  Saturation : Saturate  UpperLimit=100  LowerLimit=-100  LinearizeAsGain=off
  in : Outport
  wires:
  In/1 -> Saturation/1
  Saturation/1 -> in/1

== system DigitalShadow/Controller/PI Controller/Saturation/Without saturation ==
  In : Inport
  in : Outport
  wires:
  In/1 -> in/1

== system DigitalShadow/Controller/Speed // position/Mechanical position to electrical angle/Angle wrapping ==
  In1 : Inport
  Constant : Constant  Value=2*pi  OutDataTypeStr=single
  Math Function : Math  Operator=mod  SignedPower=on
  θs : Outport
  wires:
  In1/1 -> Math Function/1
  Constant/1 -> Math Function/2
  Math Function/1 -> θs/1

== system DigitalShadow/Controller/Speed // position/Rotor mechanical speed/Angle derivator ==
  note: accounts for discontinuities in the measured angle
  angle : Inport
  Fcn : Fcn  Expr=u(1)+2*pi*((u(1)-u(2))<-pi)-2*pi*((u(1)-u(2)>pi))
  Mux : Mux  Inputs=2
  Sum : Sum  Inputs=|+-
  Unit Delay : UnitDelay  SampleTime=CTRLPERIOD(1)  HasFrameUpgradeWarning=on
  Weighted Sample Time : SampleTimeMath  TsampMathOp=/
  speed : Outport
  wires:
  Fcn/1 -> Sum/1
  Unit Delay/1 -> Mux/2, Sum/2
  Mux/1 -> Fcn/1
  angle/1 -> Unit Delay/1, Mux/1
  Sum/1 -> Weighted Sample Time/1
  Weighted Sample Time/1 -> speed/1

== system DigitalShadow/Controller/Speed // position/Rotor mechanical speed/Low-pass filter ==
  note: fc = cut-off frequency (from mask)
      | Ts = sample time
      | tc = 1 / (2*pi*fc);
      | alpha = Ts / (tc + Ts);
  in : Inport
  reset : Inport  Port=2
  Compute alpha : Subsystem
  Constant : Constant  Value=100
  IIR : Subsystem  mask(Basic IIR LPF filter){}
      mask help:
      | The output is computed as:
      | y[k] = G * y[k-1] + (1-G) * u[k]
  out : Outport
  wires:
  in/1 -> IIR/2(u)
  reset/1 -> IIR/3(reset)
  Compute alpha/1(α) -> IIR/1(α)
  IIR/1(y) -> out/1
  Constant/1 -> Compute alpha/1(fc)

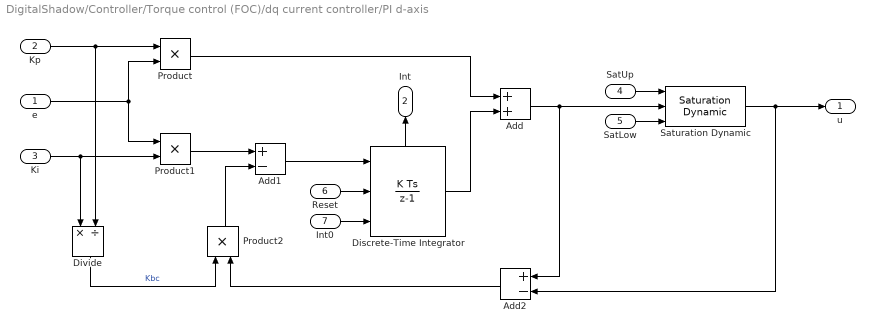
== system DigitalShadow/Controller/Torque control (FOC)/dq current controller/PI d-axis ==
  e : Inport
  Kp : Inport  Port=2
  Ki : Inport  Port=3
  SatUp : Inport  Port=4
  SatLow : Inport  Port=5
  Reset : Inport  Port=6
  Int0 : Inport  Port=7
  Add : Sum
  Add1 : Sum  Inputs=+-
  Add2 : Sum  Inputs=+-
  Discrete-Time Integrator : DiscreteIntegrator  ExternalReset=level  InitialConditionSource=external  SampleTime=-1  ShowStatePort=on  ICPrevOutput=DiscIntNeverNeededParam  ICPrevScaledInput=DiscIntNeverNeededParam
  Divide : Product  Inputs=*/
  Product : Product
  Product1 : Product
  Product2 : Product
  Saturation Dynamic : simulink/Discontinuities/Saturation Dynamic  OutMin=[]  OutMax=[]  OutDataTypeStr=Inherit: Same as second input  OutDataType=fixdt(1, 16)  OutScaling=2^-10  DoSatur=off
  u : Outport
  Int : Outport  Port=2
  wires:
  Kp/1 -> Divide/2, Product/1
  e/1 -> Product1/1, Product/2
  Product1/1 -> Add1/1
  Add1/1 -> Discrete-Time Integrator/1
  Product/1 -> Add/1
  Discrete-Time Integrator/1 -> Add/2
  Add/1 -> Add2/1, Saturation Dynamic/2
  Saturation Dynamic/1 -> Add2/2, u/1
  Product2/1 -> Add1/2
  Add2/1 -> Product2/2
  Ki/1 -> Divide/1, Product1/2
  Divide/1 -> Product2/1  "Kbc"
  SatLow/1 -> Saturation Dynamic/3
  SatUp/1 -> Saturation Dynamic/1
  Reset/1 -> Discrete-Time Integrator/2
  Int0/1 -> Discrete-Time Integrator/3
  Discrete-Time Integrator/State -> Int/1

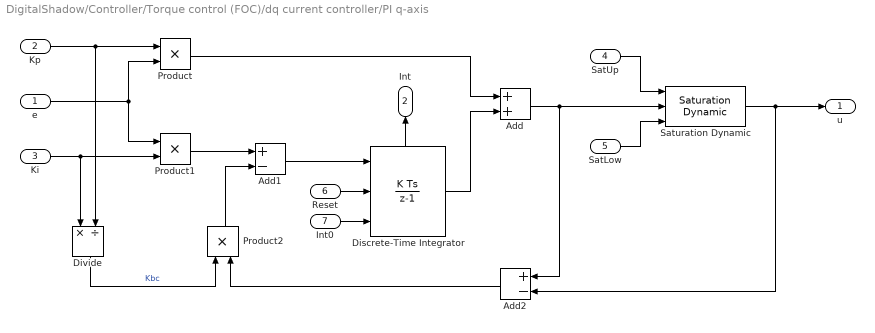
== system DigitalShadow/Controller/Torque control (FOC)/dq current controller/PI q-axis ==
  e : Inport
  Kp : Inport  Port=2
  Ki : Inport  Port=3
  SatUp : Inport  Port=4
  SatLow : Inport  Port=5
  Reset : Inport  Port=6
  Int0 : Inport  Port=7
  Add : Sum
  Add1 : Sum  Inputs=+-
  Add2 : Sum  Inputs=+-
  Discrete-Time Integrator : DiscreteIntegrator  ExternalReset=level  InitialConditionSource=external  SampleTime=-1  ShowStatePort=on  ICPrevOutput=DiscIntNeverNeededParam  ICPrevScaledInput=DiscIntNeverNeededParam
  Divide : Product  Inputs=*/
  Product : Product
  Product1 : Product
  Product2 : Product
  Saturation Dynamic : simulink/Discontinuities/Saturation Dynamic  OutMin=[]  OutMax=[]  OutDataTypeStr=Inherit: Same as second input  OutDataType=fixdt(1, 16)  OutScaling=2^-10  DoSatur=off
  u : Outport
  Int : Outport  Port=2
  wires:
  Kp/1 -> Divide/2, Product/1
  e/1 -> Product1/1, Product/2
  Product1/1 -> Add1/1
  Add1/1 -> Discrete-Time Integrator/1
  Product/1 -> Add/1
  Discrete-Time Integrator/1 -> Add/2
  Add/1 -> Add2/1, Saturation Dynamic/2
  Saturation Dynamic/1 -> Add2/2, u/1
  Product2/1 -> Add1/2
  Add2/1 -> Product2/2
  Ki/1 -> Divide/1, Product1/2
  Divide/1 -> Product2/1  "Kbc"
  SatLow/1 -> Saturation Dynamic/3
  SatUp/1 -> Saturation Dynamic/1
  Reset/1 -> Discrete-Time Integrator/2
  Int0/1 -> Discrete-Time Integrator/3
  Discrete-Time Integrator/State -> Int/1

== system DigitalShadow/Controller/Speed // position/Rotor mechanical speed/Low-pass filter/Compute alpha ==
  fc : Inport
  Fcn1 : Fcn  Expr=1/(2*pi*u(1))
  Fcn2 : Fcn  Expr=1/u(1)
  Weighted Sample Time1 : SampleTimeMath
  Weighted Sample Time2 : SampleTimeMath  TsampMathOp=*
  α : Outport
  wires:
  Fcn1/1 -> Weighted Sample Time1/1  "tc"
  fc/1 -> Fcn1/1
  Weighted Sample Time2/1 -> α/1  "Ts/(tc+Ts)"
  Fcn2/1 -> Weighted Sample Time2/1  "1/(tc+Ts)"
  Weighted Sample Time1/1 -> Fcn2/1  "tc+Ts"

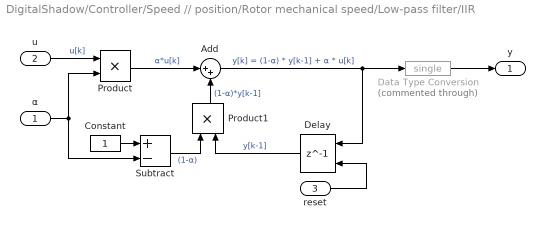
== system DigitalShadow/Controller/Speed // position/Rotor mechanical speed/Low-pass filter/IIR ==
  α : Inport
  u : Inport  Port=2
  reset : Inport  Port=3
  Add : Sum  Inputs=|++
  Constant : Constant  OutDataTypeStr=Inherit: Inherit via back propagation
  Data Type Conversion : DataTypeConversion  Commented=through  OutDataTypeStr=single  SaturateOnIntegerOverflow=off  RndMeth=Floor
  Delay : Delay  DelayLength=1  ExternalReset=Level hold
      settings: InputPortMap=u0,r5
  Product : Product
  Product1 : Product
  Subtract : Sum  Inputs=+-
  y : Outport
  wires:
  u/1 -> Product/1  "u[k]"
  Subtract/1 -> Product1/1  "(1-α)"
  α/1 -> Subtract/2, Product/2
  Constant/1 -> Subtract/1
  reset/1 -> Delay/2
  Delay/1 -> Product1/2  "y[k-1]"
  Product/1 -> Add/1  "α*u[k]"
  Product1/1 -> Add/2  "(1-α)*y[k-1]"
  Add/1 -> Data Type Conversion/1, Delay/1  "y[k] = (1-α) * y[k-1] + α * u[k]"
  Data Type Conversion/1 -> y/1
